simulink model "EXP04_Files"  (R2020a)
settings: Solver=ode4  StartTime=0.0  StopTime=100.0  FixedStep=1e-3  RelTol=1e-3
values from neighbouring files (symbols this model uses):
  g = 9.81    [EXP04_Init_file.m]
  Kd = 15    [EXP04_Init_file.m]
  Ki = 10    [EXP04_Init_file.m]
  Kp = 50    [EXP04_Init_file.m]
  l1 = 1    [EXP04_Init_file.m]
  lc1 = l1/2    (= 0.5)    [EXP04_Init_file.m]
  lc2 = l2/2    (= 0.5)    [EXP04_Init_file.m]
  m1 = 10    [EXP04_Init_file.m]
  m2 = 7    [EXP04_Init_file.m]
  tau_down = -200    [EXP04_Init_file.m]
  tau_up = 200    [EXP04_Init_file.m]
undefined symbols (not defined in the file or in its folder): I1zz, I2zz
settings Model: Creator=baradaran  LastModifiedBy=User
settings DataIOCC: ReturnWorkspaceOutputs=off
settings DebuggingCC: ArithmeticOperatorsInVariantConditions=warning
settings SFSimCC: SimUseLocalCustomCode=off  CustomCodeUndefinedFunction=UseInterfaceOnly
settings RTWCC: RTWUseLocalCustomCode=off
settings CodeAppCC: StateflowObjectComments=on

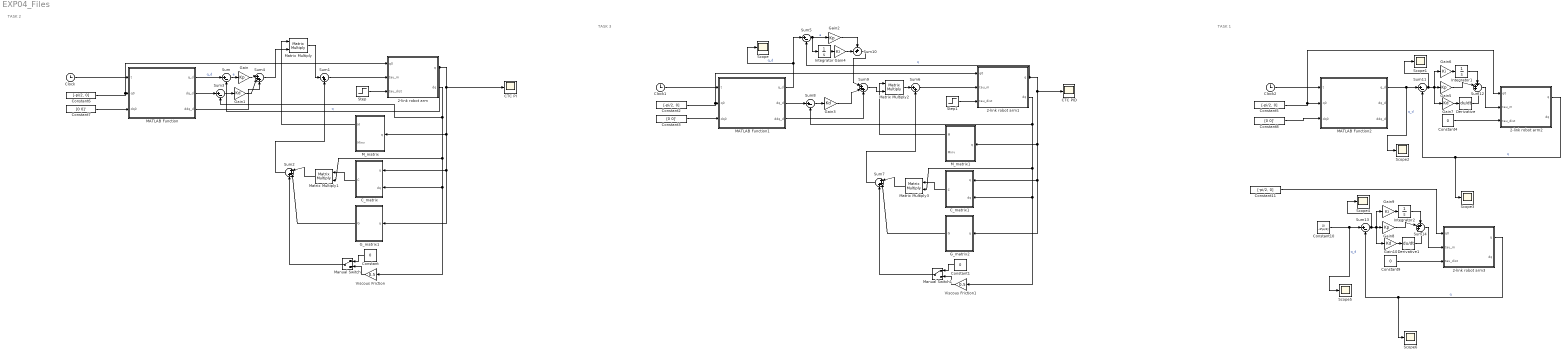
== system EXP04_Files ==
  note: TASK 2
  note: TASK 3
  note: TASK 1
  2-link robot arm : Subsystem
  2-link robot arm1 : Subsystem
  2-link robot arm2 : Subsystem
  2-link robot arm3 : Subsystem
  CTC PI : Scope
  CTC PID : Scope
  C_matrix : MATLAB Function  TreatAsAtomicUnit=on
  C_matrix1 : MATLAB Function  TreatAsAtomicUnit=on
  Clock : Clock
  Clock1 : Clock
  Clock2 : Clock
  Constant{,1,4,9} (4 alike) : Constant  Value=0
  Constant10 : Constant  Value=[0 -3*pi/4]
  Constant{2,5..6,11} (4 alike) : Constant  Value=[-pi/2, 0]
  Constant3 : Constant  Value=[0 0]'
  Constant7 : Constant  Value=[0 0]'
  Constant8 : Constant  Value=[0 0]'
  Derivative : Derivative
  Derivative1 : Derivative
  G_matrix1 : MATLAB Function  TreatAsAtomicUnit=on
  G_matrix2 : MATLAB Function  TreatAsAtomicUnit=on
  Gain{,2,5,8} (4 alike) : Gain  Gain=Kp
  Gain{1,3,7,10} (4 alike) : Gain  Gain=Kd
  Gain4 : Gain  Gain=Ki
  Gain6 : Gain  Gain=Ki
  Gain9 : Gain  Gain=Ki
  Integrator : Integrator
  Integrator1 : Integrator
  Integrator2 : Integrator
  MATLAB Function : MATLAB Function  TreatAsAtomicUnit=on
  MATLAB Function1 : MATLAB Function  TreatAsAtomicUnit=on
  MATLAB Function2 : MATLAB Function  TreatAsAtomicUnit=on
  M_matrix : MATLAB Function  TreatAsAtomicUnit=on
  M_matrix1 : MATLAB Function  TreatAsAtomicUnit=on
  Manual Switch : ManualSwitch
  Manual Switch1 : ManualSwitch
  Matrix Multiply{,1..3} (4 alike) : Product  Multiplication=Matrix(*)
  Scope{,1..6} (7 alike) : Scope
  Step : Step  Time=5  After=10  SampleTime=0
  Step1 : Step  Time=5  After=10  SampleTime=0
  Sum{,3,5,8,11,13} (6 alike) : Sum  Inputs=|+-
  Sum1 : Sum  Inputs=|++
  Sum10 : Sum  Inputs=++|
  Sum12 : Sum  Inputs=+++|
  Sum14 : Sum  Inputs=+++|
  Sum{2,4,7,9} (4 alike) : Sum  Inputs=|+++
  Sum6 : Sum  Inputs=|++
  Viscous Friction : Gain  Gain=0.5
  Viscous Friction1 : Gain  Gain=0.5
  wires:
  Constant6/1 -> 2-link robot arm/1(q0), MATLAB Function/2(q0)
  Clock/1 -> MATLAB Function/1(t)
  Constant7/1 -> MATLAB Function/3(dq0)
  Step/1 -> 2-link robot arm/3(tau_dist)
  Constant/1 -> Manual Switch/1
  Viscous Friction/1 -> Manual Switch/2
  2-link robot arm/1("q ") -> Sum/2, CTC PI/1, M_matrix/1(q), C_matrix/1(q), G_matrix1/1(q)  "q"
  2-link robot arm/2("dq ") -> Sum3/2, Viscous Friction/1, C_matrix/2(dq), Matrix Multiply1/2
  MATLAB Function/1(q_d) -> Sum/1  "q_d"
  G_matrix1/1(G) -> Sum2/2
  Matrix Multiply1/1 -> Sum2/1
  Manual Switch/1 -> Sum2/3
  Sum2/1 -> Sum1/2
  Matrix Multiply/1 -> Sum1/1
  Sum1/1 -> 2-link robot arm/2(tau_m)
  M_matrix/1(M) -> Matrix Multiply/1
  C_matrix/1(C) -> Matrix Multiply1/1
  Sum/1 -> Gain/1  "e"
  MATLAB Function/2(dq_d) -> Sum3/1
  Sum3/1 -> Gain1/1
  Sum4/1 -> Matrix Multiply/2
  Gain/1 -> Sum4/1
  Gain1/1 -> Sum4/2
  MATLAB Function/3(ddq_d) -> Sum4/3
  2-link robot arm1/2("dq ") -> Sum8/2, Viscous Friction1/1, C_matrix1/2(dq), Matrix Multiply3/2
  MATLAB Function1/2(dq_d) -> Sum8/1
  Matrix Multiply3/1 -> Sum7/1
  Matrix Multiply2/1 -> Sum6/1
  2-link robot arm1/1("q ") -> Sum5/2, CTC PID/1, M_matrix1/1(q), C_matrix1/1(q), G_matrix2/1(q)  "q"
  C_matrix1/1(C) -> Matrix Multiply3/1
  M_matrix1/1(M) -> Matrix Multiply2/1
  Sum7/1 -> Sum6/2
  Constant1/1 -> Manual Switch1/1
  Viscous Friction1/1 -> Manual Switch1/2
  MATLAB Function1/3(ddq_d) -> Sum9/3
  Gain3/1 -> Sum9/2
  Manual Switch1/1 -> Sum7/3
  Sum6/1 -> 2-link robot arm1/2(tau_m)
  Sum9/1 -> Matrix Multiply2/2
  Step1/1 -> 2-link robot arm1/3(tau_dist)
  Constant3/1 -> MATLAB Function1/3(dq0)
  MATLAB Function1/1(q_d) -> Sum5/1, Scope/1  "q_d"
  Clock1/1 -> MATLAB Function1/1(t)
  Sum8/1 -> Gain3/1
  Sum5/1 -> Integrator/1, Gain2/1  "e"
  Constant2/1 -> 2-link robot arm1/1(q0), MATLAB Function1/2(q0)
  G_matrix2/1(G) -> Sum7/2
  Integrator/1 -> Gain4/1
  Gain4/1 -> Sum10/2
  Gain2/1 -> Sum10/1
  Sum10/1 -> Sum9/1
  Clock2/1 -> MATLAB Function2/1(t)
  Constant8/1 -> MATLAB Function2/3(dq0)
  Constant4/1 -> 2-link robot arm2/3(tau_dist)
  2-link robot arm2/1("q ") -> Scope3/1, Sum11/2  "q"
  Sum11/1 -> Scope1/1, Gain7/1, Gain5/1, Gain6/1
  MATLAB Function2/1(q_d) -> Scope2/1, Sum11/1  "q_d"
  Gain6/1 -> Integrator1/1
  Gain7/1 -> Derivative/1
  Integrator1/1 -> Sum12/1
  Gain5/1 -> Sum12/2
  Derivative/1 -> Sum12/3
  Sum12/1 -> 2-link robot arm2/2(tau_m)
  Constant5/1 -> 2-link robot arm2/1(q0), MATLAB Function2/2(q0)
  Gain8/1 -> Sum14/2
  Constant10/1 -> Scope5/1, Sum13/1  "q_d"
  Gain9/1 -> Integrator2/1
  Sum13/1 -> Scope4/1, Gain10/1, Gain8/1, Gain9/1
  Sum14/1 -> 2-link robot arm3/2(tau_m)
  2-link robot arm3/1("q ") -> Scope6/1, Sum13/2  "q"
  Integrator2/1 -> Sum14/1
  Gain10/1 -> Derivative1/1
  Derivative1/1 -> Sum14/3
  Constant11/1 -> 2-link robot arm3/1(q0)
  Constant9/1 -> 2-link robot arm3/3(tau_dist)

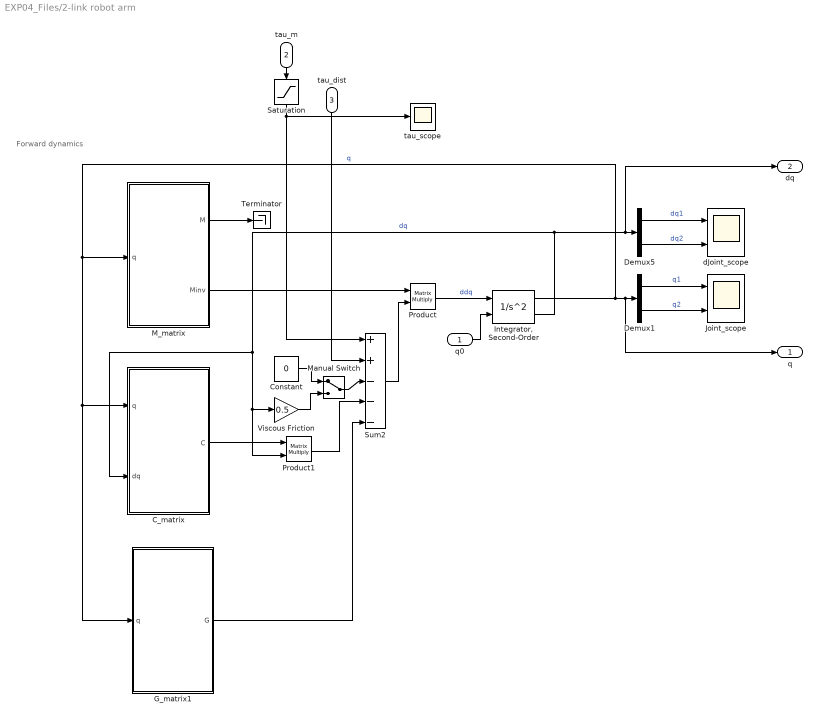
== system EXP04_Files/2-link robot arm ==
  note: Forward dynamics
  q0 : Inport
  tau_m : Inport  Port=2
  tau_dist : Inport  Port=3
  C_matrix : MATLAB Function  TreatAsAtomicUnit=on
  Constant : Constant  Value=0
  Demux1 : Demux  Outputs=2
  Demux5 : Demux  Outputs=2
  G_matrix1 : MATLAB Function  TreatAsAtomicUnit=on
  "Integrator, Second-Order" : SecondOrderIntegrator  ICSourceX=external
  Joint_scope : Scope  NumInputPorts=2
  M_matrix : MATLAB Function  TreatAsAtomicUnit=on
  Manual Switch : ManualSwitch
  Product : Product  Multiplication=Matrix(*)
  Product1 : Product  Multiplication=Matrix(*)
  Saturation : Saturate  UpperLimit=tau_up  LowerLimit=tau_down
  Sum2 : Sum  Inputs=++|---
  Terminator : Terminator
  Viscous Friction : Gain  Gain=0.5
  dJoint_scope : Scope  NumInputPorts=2
  tau_scope : Scope
  "q " : Outport
  "dq " : Outport  Port=2
  wires:
  Saturation/1 -> Sum2/1, tau_scope/1
  q0/1 -> "Integrator, Second-Order"/2
  tau_dist/1 -> Sum2/2
  tau_m/1 -> Saturation/1
  Manual Switch/1 -> Sum2/3
  Product1/1 -> Sum2/4
  G_matrix1/1(G) -> Sum2/5
  Product/1 -> "Integrator, Second-Order"/1  "ddq"
  M_matrix/1(M) -> Terminator/1
  Viscous Friction/1 -> Manual Switch/2
  Constant/1 -> Manual Switch/1
  Sum2/1 -> Product/2
  Demux5/2 -> dJoint_scope/2  "dq2"
  M_matrix/2(Minv) -> Product/1
  "Integrator, Second-Order"/1 -> Demux1/1, "q "/1, M_matrix/1(q), C_matrix/1(q), G_matrix1/1(q)  "q"
  C_matrix/1(C) -> Product1/1
  Demux5/1 -> dJoint_scope/1  "dq1"
  "Integrator, Second-Order"/2 -> Demux5/1, "dq "/1, Viscous Friction/1, Product1/2, C_matrix/2(dq)  "dq"
  Demux1/2 -> Joint_scope/2  "q2"
  Demux1/1 -> Joint_scope/1  "q1"

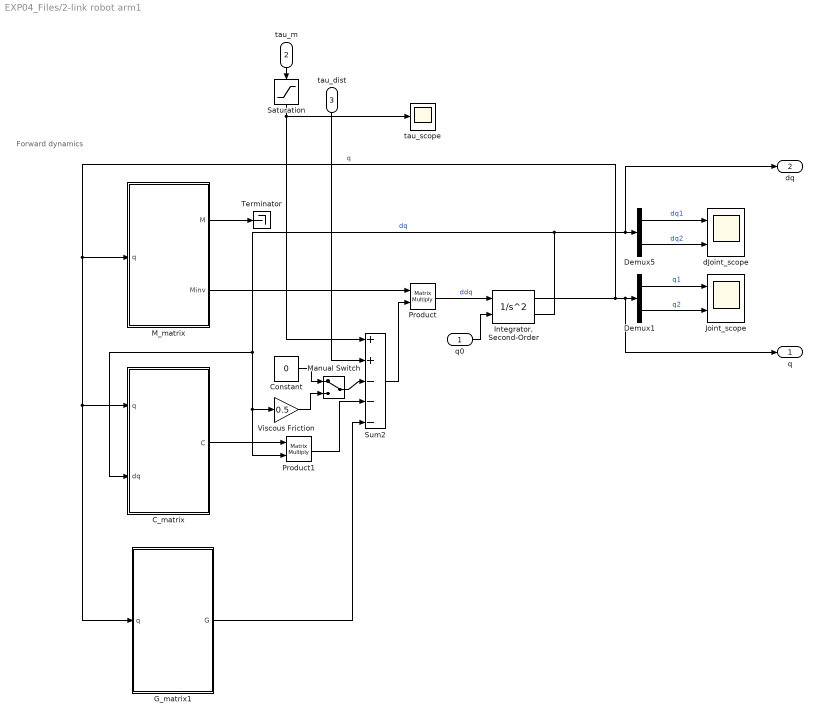
== system EXP04_Files/2-link robot arm1 ==
  note: Forward dynamics
  q0 : Inport
  tau_m : Inport  Port=2
  tau_dist : Inport  Port=3
  C_matrix : MATLAB Function  TreatAsAtomicUnit=on
  Constant : Constant  Value=0
  Demux1 : Demux  Outputs=2
  Demux5 : Demux  Outputs=2
  G_matrix1 : MATLAB Function  TreatAsAtomicUnit=on
  "Integrator, Second-Order" : SecondOrderIntegrator  ICSourceX=external
  Joint_scope : Scope  NumInputPorts=2
  M_matrix : MATLAB Function  TreatAsAtomicUnit=on
  Manual Switch : ManualSwitch
  Product : Product  Multiplication=Matrix(*)
  Product1 : Product  Multiplication=Matrix(*)
  Saturation : Saturate  UpperLimit=tau_up  LowerLimit=tau_down
  Sum2 : Sum  Inputs=++|---
  Terminator : Terminator
  Viscous Friction : Gain  Gain=0.5
  dJoint_scope : Scope  NumInputPorts=2
  tau_scope : Scope
  "q " : Outport
  "dq " : Outport  Port=2
  wires:
  Saturation/1 -> Sum2/1, tau_scope/1
  q0/1 -> "Integrator, Second-Order"/2
  tau_dist/1 -> Sum2/2
  tau_m/1 -> Saturation/1
  Manual Switch/1 -> Sum2/3
  Product1/1 -> Sum2/4
  G_matrix1/1(G) -> Sum2/5
  Product/1 -> "Integrator, Second-Order"/1  "ddq"
  M_matrix/1(M) -> Terminator/1
  Viscous Friction/1 -> Manual Switch/2
  Constant/1 -> Manual Switch/1
  Sum2/1 -> Product/2
  Demux5/2 -> dJoint_scope/2  "dq2"
  M_matrix/2(Minv) -> Product/1
  "Integrator, Second-Order"/1 -> Demux1/1, "q "/1, M_matrix/1(q), C_matrix/1(q), G_matrix1/1(q)  "q"
  C_matrix/1(C) -> Product1/1
  Demux5/1 -> dJoint_scope/1  "dq1"
  "Integrator, Second-Order"/2 -> Demux5/1, "dq "/1, Viscous Friction/1, Product1/2, C_matrix/2(dq)  "dq"
  Demux1/2 -> Joint_scope/2  "q2"
  Demux1/1 -> Joint_scope/1  "q1"

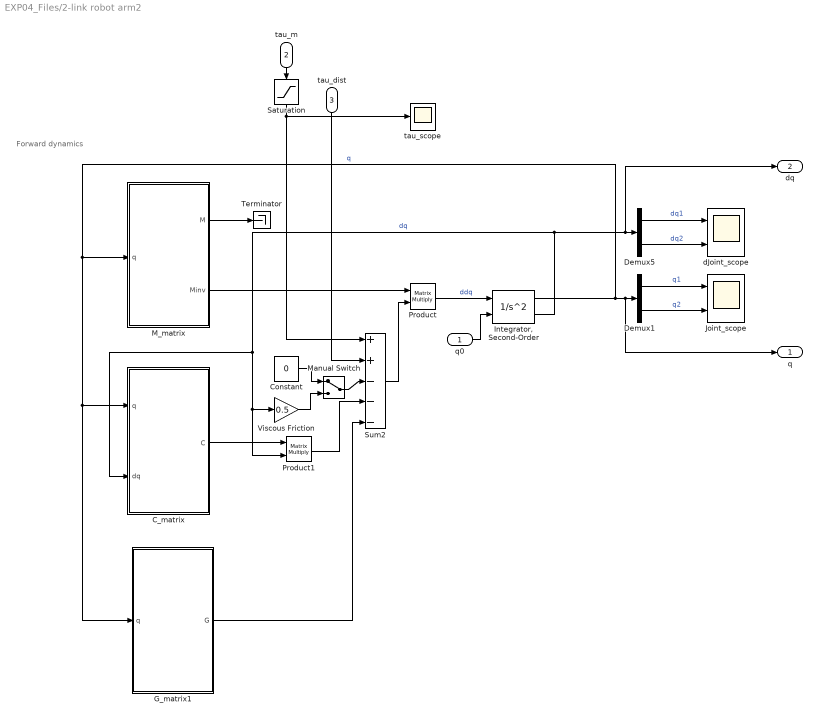
== system EXP04_Files/2-link robot arm2 ==
  note: Forward dynamics
  q0 : Inport
  tau_m : Inport  Port=2
  tau_dist : Inport  Port=3
  C_matrix : MATLAB Function  TreatAsAtomicUnit=on
  Constant : Constant  Value=0
  Demux1 : Demux  Outputs=2
  Demux5 : Demux  Outputs=2
  G_matrix1 : MATLAB Function  TreatAsAtomicUnit=on
  "Integrator, Second-Order" : SecondOrderIntegrator  ICSourceX=external
  Joint_scope : Scope  NumInputPorts=2
  M_matrix : MATLAB Function  TreatAsAtomicUnit=on
  Manual Switch : ManualSwitch
  Product : Product  Multiplication=Matrix(*)
  Product1 : Product  Multiplication=Matrix(*)
  Saturation : Saturate  UpperLimit=tau_up  LowerLimit=tau_down
  Sum2 : Sum  Inputs=++|---
  Terminator : Terminator
  Viscous Friction : Gain  Gain=0.5
  dJoint_scope : Scope  NumInputPorts=2
  tau_scope : Scope
  "q " : Outport
  "dq " : Outport  Port=2
  wires:
  Saturation/1 -> Sum2/1, tau_scope/1
  q0/1 -> "Integrator, Second-Order"/2
  tau_dist/1 -> Sum2/2
  tau_m/1 -> Saturation/1
  Manual Switch/1 -> Sum2/3
  Product1/1 -> Sum2/4
  G_matrix1/1(G) -> Sum2/5
  Product/1 -> "Integrator, Second-Order"/1  "ddq"
  M_matrix/1(M) -> Terminator/1
  Viscous Friction/1 -> Manual Switch/2
  Constant/1 -> Manual Switch/1
  Sum2/1 -> Product/2
  Demux5/2 -> dJoint_scope/2  "dq2"
  M_matrix/2(Minv) -> Product/1
  "Integrator, Second-Order"/1 -> Demux1/1, "q "/1, M_matrix/1(q), C_matrix/1(q), G_matrix1/1(q)  "q"
  C_matrix/1(C) -> Product1/1
  Demux5/1 -> dJoint_scope/1  "dq1"
  "Integrator, Second-Order"/2 -> Demux5/1, "dq "/1, Viscous Friction/1, Product1/2, C_matrix/2(dq)  "dq"
  Demux1/2 -> Joint_scope/2  "q2"
  Demux1/1 -> Joint_scope/1  "q1"

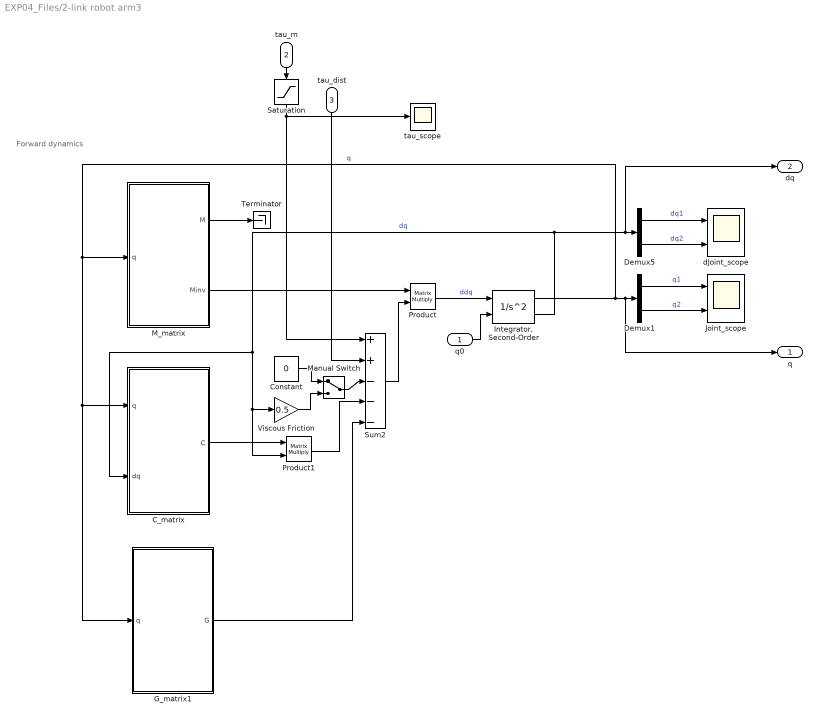
== system EXP04_Files/2-link robot arm3 ==
  note: Forward dynamics
  q0 : Inport
  tau_m : Inport  Port=2
  tau_dist : Inport  Port=3
  C_matrix : MATLAB Function  TreatAsAtomicUnit=on
  Constant : Constant  Value=0
  Demux1 : Demux  Outputs=2
  Demux5 : Demux  Outputs=2
  G_matrix1 : MATLAB Function  TreatAsAtomicUnit=on
  "Integrator, Second-Order" : SecondOrderIntegrator  ICSourceX=external
  Joint_scope : Scope  NumInputPorts=2
  M_matrix : MATLAB Function  TreatAsAtomicUnit=on
  Manual Switch : ManualSwitch
  Product : Product  Multiplication=Matrix(*)
  Product1 : Product  Multiplication=Matrix(*)
  Saturation : Saturate  UpperLimit=tau_up  LowerLimit=tau_down
  Sum2 : Sum  Inputs=++|---
  Terminator : Terminator
  Viscous Friction : Gain  Gain=0.5
  dJoint_scope : Scope  NumInputPorts=2
  tau_scope : Scope
  "q " : Outport
  "dq " : Outport  Port=2
  wires:
  Saturation/1 -> Sum2/1, tau_scope/1
  q0/1 -> "Integrator, Second-Order"/2
  tau_dist/1 -> Sum2/2
  tau_m/1 -> Saturation/1
  Manual Switch/1 -> Sum2/3
  Product1/1 -> Sum2/4
  G_matrix1/1(G) -> Sum2/5
  Product/1 -> "Integrator, Second-Order"/1  "ddq"
  M_matrix/1(M) -> Terminator/1
  Viscous Friction/1 -> Manual Switch/2
  Constant/1 -> Manual Switch/1
  Sum2/1 -> Product/2
  Demux5/2 -> dJoint_scope/2  "dq2"
  M_matrix/2(Minv) -> Product/1
  "Integrator, Second-Order"/1 -> Demux1/1, "q "/1, M_matrix/1(q), C_matrix/1(q), G_matrix1/1(q)  "q"
  C_matrix/1(C) -> Product1/1
  Demux5/1 -> dJoint_scope/1  "dq1"
  "Integrator, Second-Order"/2 -> Demux5/1, "dq "/1, Viscous Friction/1, Product1/2, C_matrix/2(dq)  "dq"
  Demux1/2 -> Joint_scope/2  "q2"
  Demux1/1 -> Joint_scope/1  "q1"

== matlab function EXP04_Files/G_matrix2 ==
  data: G output; q input; g parameter; l1 parameter; lc1 parameter; lc2 parameter; m1 parameter; m2 parameter
function G = G_matrix(q, g, l1, lc1, lc2, m1, m2)
%#codegen

%    This function was generated by the Symbolic Math Toolbox version 8.3.
%    05-Nov-2019 15:18:30
q1 = q(1);
q2 = q(2);
t2 = cos(q1);
t3 = q1+q2;
t4 = cos(t3);
G = [g.*m2.*(l1.*t2+lc2.*t4)+g.*lc1.*m1.*t2;g.*lc2.*m2.*t4];

== matlab function EXP04_Files/MATLAB Function1 ==
  data: t input; q_d output; q0 input; dq0 input; dq_d output; ddq_d output
function [q_d, dq_d, ddq_d] = desired_traj(t,q0,dq0)
    A = 5*[1; 1];
    B = 5*[1; 1];
    w = 2*pi*1;

    q_d   = -A./w^2*sin(w*t) -B./(2*w)^2*cos(2*w*t) + dq0*t + q0;
    dq_d  = -A./w*cos(w*t) + B./(2*w)*sin(2*w*t) + dq0;
    ddq_d = A*sin(w*t) + B*cos(2*w*t);
end

== matlab function EXP04_Files/MATLAB Function ==
  data: t input; q_d output; q0 input; dq0 input; dq_d output; ddq_d output
function [q_d, dq_d, ddq_d] = desired_traj(t,q0,dq0)
    A = 5*[1; 1];
    B = 5*[1; 1];
    w = 2*pi*1;

    q_d   = -A./w^2*sin(w*t) -B./(2*w)^2*cos(2*w*t) + dq0*t + q0;
    dq_d  = -A./w*cos(w*t) + B./(2*w)*sin(2*w*t) + dq0;
    ddq_d = A*sin(w*t) + B*cos(2*w*t);
end

== matlab function EXP04_Files/M_matrix1 ==
  data: M output; q input; I1zz parameter; I2zz parameter; l1 parameter; lc1 parameter; lc2 parameter; m1 parameter; m2 parameter; Minv output
function [M, Minv] = M_matrix(q, I1zz, I2zz, l1, lc1, lc2, m1, m2)
%#codegen

%    This function was generated by the Symbolic Math Toolbox version 8.3.
%    05-Nov-2019 15:18:29
q1 = q(1);
q2 = q(2);
t2 = cos(q2);
t3 = lc2.^2;
t4 = m2.*t3;
t5 = l1.*lc2.*m2.*t2;
t6 = I2zz+t4+t5;
M = reshape([I1zz+t5+t6+l1.^2.*m2+lc1.^2.*m1,t6,t6,I2zz+t4],[2,2]);
Minv = pinv(M);

== matlab function EXP04_Files/2-link robot arm2/C_matrix ==
  data: q input; C output; dq input; l1 parameter; lc2 parameter; m2 parameter
function C = C_matrix(q,dq, l1, lc2, m2)
%#codegen

%    This function was generated by the Symbolic Math Toolbox version 8.3.
%    05-Nov-2019 15:18:30
q1 = q(1);
q2 = q(2);
dq1 = dq(1);
dq2 = dq(2);
t2 = sin(q2);
C = reshape([-dq2.*l1.*lc2.*m2.*t2,dq1.*l1.*lc2.*m2.*t2,-l1.*lc2.*m2.*t2.*(dq1+dq2),0.0],[2,2]);

== matlab function EXP04_Files/M_matrix ==
  data: M output; q input; I1zz parameter; I2zz parameter; l1 parameter; lc1 parameter; lc2 parameter; m1 parameter; m2 parameter; Minv output
function [M, Minv] = M_matrix(q, I1zz, I2zz, l1, lc1, lc2, m1, m2)
%#codegen

%    This function was generated by the Symbolic Math Toolbox version 8.3.
%    05-Nov-2019 15:18:29
q1 = q(1);
q2 = q(2);
t2 = cos(q2);
t3 = lc2.^2;
t4 = m2.*t3;
t5 = l1.*lc2.*m2.*t2;
t6 = I2zz+t4+t5;
M = reshape([I1zz+t5+t6+l1.^2.*m2+lc1.^2.*m1,t6,t6,I2zz+t4],[2,2]);
Minv = pinv(M);

== matlab function EXP04_Files/2-link robot arm2/G_matrix1 ==
  data: G output; q input; g parameter; l1 parameter; lc1 parameter; lc2 parameter; m1 parameter; m2 parameter
function G = G_matrix(q, g, l1, lc1, lc2, m1, m2)
%#codegen

%    This function was generated by the Symbolic Math Toolbox version 8.3.
%    05-Nov-2019 15:18:30
q1 = q(1);
q2 = q(2);
t2 = cos(q1);
t3 = q1+q2;
t4 = cos(t3);
G = [g.*m2.*(l1.*t2+lc2.*t4)+g.*lc1.*m1.*t2;g.*lc2.*m2.*t4];

== matlab function EXP04_Files/2-link robot arm2/M_matrix ==
  data: M output; q input; I1zz parameter; I2zz parameter; l1 parameter; lc1 parameter; lc2 parameter; m1 parameter; m2 parameter; Minv output
function [M, Minv] = M_matrix(q, I1zz, I2zz, l1, lc1, lc2, m1, m2)
%#codegen

%    This function was generated by the Symbolic Math Toolbox version 8.3.
%    05-Nov-2019 15:18:29
q1 = q(1);
q2 = q(2);
t2 = cos(q2);
t3 = lc2.^2;
t4 = m2.*t3;
t5 = l1.*lc2.*m2.*t2;
t6 = I2zz+t4+t5;
M = reshape([I1zz+t5+t6+l1.^2.*m2+lc1.^2.*m1,t6,t6,I2zz+t4],[2,2]);
Minv = pinv(M);

== matlab function EXP04_Files/2-link robot arm3/C_matrix ==
  data: q input; C output; dq input; l1 parameter; lc2 parameter; m2 parameter
function C = C_matrix(q,dq, l1, lc2, m2)
%#codegen

%    This function was generated by the Symbolic Math Toolbox version 8.3.
%    05-Nov-2019 15:18:30
q1 = q(1);
q2 = q(2);
dq1 = dq(1);
dq2 = dq(2);
t2 = sin(q2);
C = reshape([-dq2.*l1.*lc2.*m2.*t2,dq1.*l1.*lc2.*m2.*t2,-l1.*lc2.*m2.*t2.*(dq1+dq2),0.0],[2,2]);

== matlab function EXP04_Files/2-link robot arm3/G_matrix1 ==
  data: G output; q input; g parameter; l1 parameter; lc1 parameter; lc2 parameter; m1 parameter; m2 parameter
function G = G_matrix(q, g, l1, lc1, lc2, m1, m2)
%#codegen

%    This function was generated by the Symbolic Math Toolbox version 8.3.
%    05-Nov-2019 15:18:30
q1 = q(1);
q2 = q(2);
t2 = cos(q1);
t3 = q1+q2;
t4 = cos(t3);
G = [g.*m2.*(l1.*t2+lc2.*t4)+g.*lc1.*m1.*t2;g.*lc2.*m2.*t4];

== matlab function EXP04_Files/MATLAB Function2 ==
  data: t input; q_d output; q0 input; dq0 input; dq_d output; ddq_d output
function [q_d, dq_d, ddq_d] = desired_traj(t,q0,dq0)
    A = 5*[1; 1];
    B = 5*[1; 1];
    w = 2*pi*1;

    q_d   = -A./w^2*sin(w*t) -B./(2*w)^2*cos(2*w*t) + dq0*t + q0;
    dq_d  = -A./w*cos(w*t) + B./(2*w)*sin(2*w*t) + dq0;
    ddq_d = A*sin(w*t) + B*cos(2*w*t);
end

== matlab function EXP04_Files/2-link robot arm3/M_matrix ==
  data: M output; q input; I1zz parameter; I2zz parameter; l1 parameter; lc1 parameter; lc2 parameter; m1 parameter; m2 parameter; Minv output
function [M, Minv] = M_matrix(q, I1zz, I2zz, l1, lc1, lc2, m1, m2)
%#codegen

%    This function was generated by the Symbolic Math Toolbox version 8.3.
%    05-Nov-2019 15:18:29
q1 = q(1);
q2 = q(2);
t2 = cos(q2);
t3 = lc2.^2;
t4 = m2.*t3;
t5 = l1.*lc2.*m2.*t2;
t6 = I2zz+t4+t5;
M = reshape([I1zz+t5+t6+l1.^2.*m2+lc1.^2.*m1,t6,t6,I2zz+t4],[2,2]);
Minv = pinv(M);

== matlab function EXP04_Files/2-link robot arm/C_matrix ==
  data: q input; C output; dq input; l1 parameter; lc2 parameter; m2 parameter
function C = C_matrix(q,dq, l1, lc2, m2)
%#codegen

%    This function was generated by the Symbolic Math Toolbox version 8.3.
%    05-Nov-2019 15:18:30
q1 = q(1);
q2 = q(2);
dq1 = dq(1);
dq2 = dq(2);
t2 = sin(q2);
C = reshape([-dq2.*l1.*lc2.*m2.*t2,dq1.*l1.*lc2.*m2.*t2,-l1.*lc2.*m2.*t2.*(dq1+dq2),0.0],[2,2]);

== matlab function EXP04_Files/2-link robot arm/G_matrix1 ==
  data: G output; q input; g parameter; l1 parameter; lc1 parameter; lc2 parameter; m1 parameter; m2 parameter
function G = G_matrix(q, g, l1, lc1, lc2, m1, m2)
%#codegen

%    This function was generated by the Symbolic Math Toolbox version 8.3.
%    05-Nov-2019 15:18:30
q1 = q(1);
q2 = q(2);
t2 = cos(q1);
t3 = q1+q2;
t4 = cos(t3);
G = [g.*m2.*(l1.*t2+lc2.*t4)+g.*lc1.*m1.*t2;g.*lc2.*m2.*t4];

== matlab function EXP04_Files/2-link robot arm/M_matrix ==
  data: M output; q input; I1zz parameter; I2zz parameter; l1 parameter; lc1 parameter; lc2 parameter; m1 parameter; m2 parameter; Minv output
function [M, Minv] = M_matrix(q, I1zz, I2zz, l1, lc1, lc2, m1, m2)
%#codegen

%    This function was generated by the Symbolic Math Toolbox version 8.3.
%    05-Nov-2019 15:18:29
q1 = q(1);
q2 = q(2);
t2 = cos(q2);
t3 = lc2.^2;
t4 = m2.*t3;
t5 = l1.*lc2.*m2.*t2;
t6 = I2zz+t4+t5;
M = reshape([I1zz+t5+t6+l1.^2.*m2+lc1.^2.*m1,t6,t6,I2zz+t4],[2,2]);
Minv = pinv(M);

== matlab function EXP04_Files/C_matrix ==
  data: q input; C output; dq input; l1 parameter; lc2 parameter; m2 parameter
function C = C_matrix(q,dq, l1, lc2, m2)
%#codegen

%    This function was generated by the Symbolic Math Toolbox version 8.3.
%    05-Nov-2019 15:18:30
q1 = q(1);
q2 = q(2);
dq1 = dq(1);
dq2 = dq(2);
t2 = sin(q2);
C = reshape([-dq2.*l1.*lc2.*m2.*t2,dq1.*l1.*lc2.*m2.*t2,-l1.*lc2.*m2.*t2.*(dq1+dq2),0.0],[2,2]);

== matlab function EXP04_Files/G_matrix1 ==
  data: G output; q input; g parameter; l1 parameter; lc1 parameter; lc2 parameter; m1 parameter; m2 parameter
function G = G_matrix(q, g, l1, lc1, lc2, m1, m2)
%#codegen

%    This function was generated by the Symbolic Math Toolbox version 8.3.
%    05-Nov-2019 15:18:30
q1 = q(1);
q2 = q(2);
t2 = cos(q1);
t3 = q1+q2;
t4 = cos(t3);
G = [g.*m2.*(l1.*t2+lc2.*t4)+g.*lc1.*m1.*t2;g.*lc2.*m2.*t4];

== matlab function EXP04_Files/2-link robot arm1/C_matrix ==
  data: q input; C output; dq input; l1 parameter; lc2 parameter; m2 parameter
function C = C_matrix(q,dq, l1, lc2, m2)
%#codegen

%    This function was generated by the Symbolic Math Toolbox version 8.3.
%    05-Nov-2019 15:18:30
q1 = q(1);
q2 = q(2);
dq1 = dq(1);
dq2 = dq(2);
t2 = sin(q2);
C = reshape([-dq2.*l1.*lc2.*m2.*t2,dq1.*l1.*lc2.*m2.*t2,-l1.*lc2.*m2.*t2.*(dq1+dq2),0.0],[2,2]);

== matlab function EXP04_Files/2-link robot arm1/G_matrix1 ==
  data: G output; q input; g parameter; l1 parameter; lc1 parameter; lc2 parameter; m1 parameter; m2 parameter
function G = G_matrix(q, g, l1, lc1, lc2, m1, m2)
%#codegen

%    This function was generated by the Symbolic Math Toolbox version 8.3.
%    05-Nov-2019 15:18:30
q1 = q(1);
q2 = q(2);
t2 = cos(q1);
t3 = q1+q2;
t4 = cos(t3);
G = [g.*m2.*(l1.*t2+lc2.*t4)+g.*lc1.*m1.*t2;g.*lc2.*m2.*t4];

== matlab function EXP04_Files/2-link robot arm1/M_matrix ==
  data: M output; q input; I1zz parameter; I2zz parameter; l1 parameter; lc1 parameter; lc2 parameter; m1 parameter; m2 parameter; Minv output
function [M, Minv] = M_matrix(q, I1zz, I2zz, l1, lc1, lc2, m1, m2)
%#codegen

%    This function was generated by the Symbolic Math Toolbox version 8.3.
%    05-Nov-2019 15:18:29
q1 = q(1);
q2 = q(2);
t2 = cos(q2);
t3 = lc2.^2;
t4 = m2.*t3;
t5 = l1.*lc2.*m2.*t2;
t6 = I2zz+t4+t5;
M = reshape([I1zz+t5+t6+l1.^2.*m2+lc1.^2.*m1,t6,t6,I2zz+t4],[2,2]);
Minv = pinv(M);

== matlab function EXP04_Files/C_matrix1 ==
  data: q input; C output; dq input; l1 parameter; lc2 parameter; m2 parameter
function C = C_matrix(q,dq, l1, lc2, m2)
%#codegen

%    This function was generated by the Symbolic Math Toolbox version 8.3.
%    05-Nov-2019 15:18:30
q1 = q(1);
q2 = q(2);
dq1 = dq(1);
dq2 = dq(2);
t2 = sin(q2);
C = reshape([-dq2.*l1.*lc2.*m2.*t2,dq1.*l1.*lc2.*m2.*t2,-l1.*lc2.*m2.*t2.*(dq1+dq2),0.0],[2,2]);
